simulink model "Derivative"  (R2020b)
settings: Solver=VariableStepAuto  StartTime=0.0  StopTime=10.0  RelTol=1e-3
settings Model: Creator=MSI  LastModifiedBy=MSI

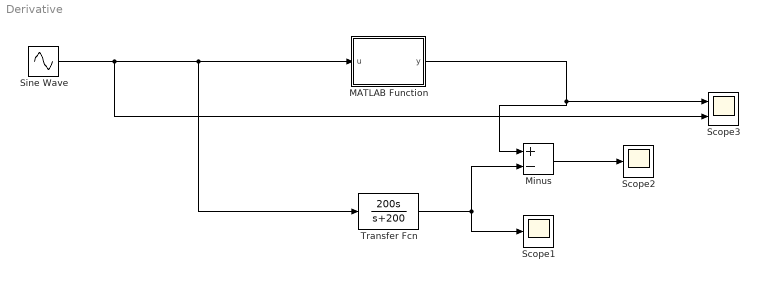
== system Derivative ==
  MATLAB Function : MATLAB Function  TreatAsAtomicUnit=on
  Minus : Sum  Inputs=+-
  Scope1 : Scope
  Scope2 : Scope
  Scope3 : Scope  NumInputPorts=2
  Sine Wave : Sin  SampleTime=0  VectorParams1D=off
  Transfer Fcn : TransferFcn  Numerator=[200 0]  Denominator=[1 200]
  wires:
  Sine Wave/1 -> Scope3/2, Transfer Fcn/1, MATLAB Function/1(u)
  MATLAB Function/1(y) -> Minus/1, Scope3/1
  Transfer Fcn/1 -> Minus/2, Scope1/1
  Minus/1 -> Scope2/1

== matlab function Derivative/MATLAB Function ==
  settings: updateMethod=DISCRETE  sampleTime=1/500
  data: u input; y output
function y = Derivative(u)

persistent Prev
persistent ept
persistent Temp
Tsample = 1/500;
nhat = 16;               % Number of samples taken/kept
P = 4/(Tsample*nhat)                 % Pole

% Initialize Temp
if isempty(Temp)
    Temp = 0;
end

% Initialize ept
if isempty(ept)
    ept = zeros(1, nhat);
    total = 0;
    for i = 1:nhat
        calc = P*exp(-P*i*Tsample);
        ept(i) = calc;
        total = total + calc;
    end
    scale = 1/(Tsample*total)
    ept = ept*scale
end

% Initialize Prev
if isempty(Prev)
    Prev = zeros(1,nhat);
end

% Compute difference
Prev(1) = (u - Temp)
y = dot(ept, Prev)

% Take a step in time
for n = 1:(nhat - 1)
    Prev(nhat + 1 - n) = Prev(nhat - n);
end

Temp = u;
end
